simulink model "uuvSim_lqr"  (R2017b)
settings: Solver=ode4  StartTime=0.0  StopTime=10.0  FixedStep=mdl.tStep  RelTol=1e-3
values from neighbouring files (symbols this model uses):
  trj_type = block.DialogPrm(1).Data    [trj_gen.m]    (also in trj_gen_mpc.m)
  waypoints = block.DialogPrm(2).Data    [trj_gen.m]    (also in trj_gen_mpc.m)
undefined symbols (not defined in the file or in its folder): ics, K, mdl, rov, Tinv, v_c
settings Model: Creator=e_anderlini  LastModifiedBy=enricoanderlini
settings CodeAppCC: StateflowObjectComments=on

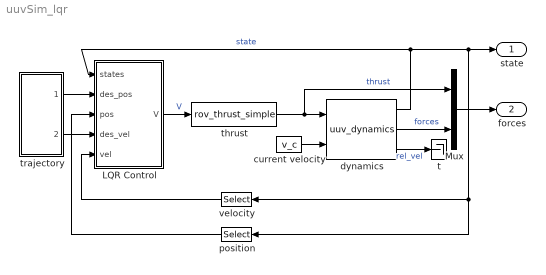
== system uuvSim_lqr ==
  LQR Control : Subsystem
  Mux : Mux  Inputs=[6,18]
  current velocity : Constant  Value=v_c
  dynamics : S-Function  FunctionName=uuv_dynamics  Parameters=rov.weight,rov.buoyancy,rov.CoG,rov.CoB,ics,rov.inv_mass',rov.M_A',rov.M_B',rov.D_l',rov.D_q'  SFunctionDeploymentMode=off  EnableBusSupport=off
  position : Selector  InputPortWidth=12  IndexOptions=Index vector (dialog)  Indices=[1 2 3 6]  OutputSizes=1
  t : Terminator
  thrust : S-Function  FunctionName=rov_thrust_simple  Parameters=rov.coeffs',rov.T'  SFunctionDeploymentMode=off  EnableBusSupport=off
  trajectory : Subsystem
  velocity : Selector  InputPortWidth=12  IndexOptions=Index vector (dialog)  Indices=[7 8 9 12]  OutputSizes=1
  state : Outport
  forces : Outport  Port=2
  wires:
  dynamics/1 -> velocity/1, position/1, state/1, LQR Control/1("states ")  "state"
  thrust/1 -> Mux/1, dynamics/1  "thrust"
  Mux/1 -> forces/1
  dynamics/2 -> Mux/2  "forces"
  LQR Control/1(V) -> thrust/1  "V"
  dynamics/3 -> t/1  "rel_vel"
  current velocity/1 -> dynamics/2
  position/1 -> LQR Control/3(pos)
  trajectory/1(trj_pos) -> LQR Control/2(des_pos)
  velocity/1 -> LQR Control/5(vel)
  trajectory/2(trj_vel) -> LQR Control/4(des_vel)

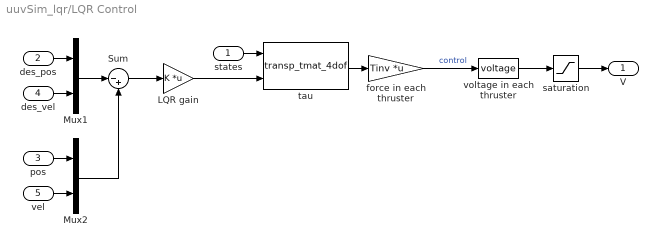
== system uuvSim_lqr/LQR Control ==
  "states " : Inport
  des_pos : Inport  Port=2
  pos : Inport  Port=3
  des_vel : Inport  Port=4
  vel : Inport  Port=5
  LQR gain : Gain  Gain=K  Multiplication=Matrix(K*u)
  Mux1 : Mux  Inputs=2
  Mux2 : Mux  Inputs=2
  Sum : Sum  Inputs=|-+
  force in each thruster : Gain  Gain=Tinv  Multiplication=Matrix(K*u)
  saturation : Saturate  UpperLimit=5  LowerLimit=-5
  tau : S-Function  FunctionName=transp_tmat_4dof  SFunctionDeploymentMode=off  EnableBusSupport=off
  voltage in each thruster : S-Function  FunctionName=voltage  Parameters=rov.inv_coeffs'  SFunctionDeploymentMode=off  EnableBusSupport=off
  V : Outport
  wires:
  force in each thruster/1 -> voltage in each thruster/1  "control"
  saturation/1 -> V/1
  LQR gain/1 -> tau/2
  des_pos/1 -> Mux1/1
  pos/1 -> Mux2/1
  "states "/1 -> tau/1
  tau/1 -> force in each thruster/1
  voltage in each thruster/1 -> saturation/1
  des_vel/1 -> Mux1/2
  vel/1 -> Mux2/2
  Mux2/1 -> Sum/2
  Mux1/1 -> Sum/1
  Sum/1 -> LQR gain/1

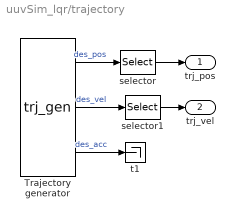
== system uuvSim_lqr/trajectory ==
  Trajectory generator : M-S-Function  FunctionName=trj_gen  Parameters=trj_type,waypoints,20,mdl.tStep
  selector : Selector  InputPortWidth=6  IndexOptions=Index vector (dialog)  Indices=[1 2 3 6]  OutputSizes=1
  selector1 : Selector  InputPortWidth=6  IndexOptions=Index vector (dialog)  Indices=[1 2 3 6]  OutputSizes=1
  t1 : Terminator
  trj_pos : Outport
  trj_vel : Outport  Port=2
  wires:
  Trajectory generator/1 -> selector/1  "des_pos"
  Trajectory generator/2 -> selector1/1  "des_vel"
  Trajectory generator/3 -> t1/1  "des_acc"
  selector/1 -> trj_pos/1
  selector1/1 -> trj_vel/1
